simulink model "CircuitB_cbv_only"  (R2024b)
settings: Solver=VariableStepAuto  StartTime=0.0  StopTime=60  MaxStep=1e-3  RelTol=1e-3
InitFcn:
  | run("circuit_B.m")
model workspace (MATLAB code in the model file):
  | %% From Project Description
  | omega_0 = 5; % [rad/sec]
  | % eta_hmM = 1;
  | % eta_vM = 1; % 100% since parallel orifices simulate this
  | 
  | %% Chosen Parameters
  | 
  | wn = 17 * 2*pi; %from datasheet
  | zeta = 1;
  | 
  | dpO_CBV = 200e5;
  | dpO_CHK = 2e5; % default 2 MRH
  | dpO_comp = 3e5; % from 5 to 10, default 3 MRH
  | 
  | pCrCBV = 216e5;
  | pCrCHK = 1.7e5; % [bar] datasheet
  | pCMP = 10e5;
  | 
  | fCO = 2; % [Hz]
  | wCO = 2*pi * fCO; % [rad/sec]
  | 
  | % alpha = 3;
  | % pCrCHK = 2;
  | 
  | %% Calculated Parameters
undefined symbols (not defined in the file): Ad_L, Ad_L_fault, alpha_cbv, g, i_pl2M, mpl, mu_eq, pcr2, Tw, Zw
libraries: nesl_utility x19, fl_lib x19, SimscapeFluids_lib x13, slpidlib x2
(part 2 of 2)

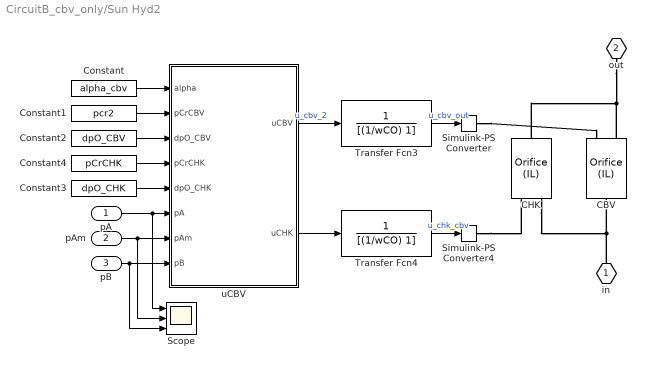
== system CircuitB_cbv_only/Sun Hyd2 ==
  pA : Inport
  pAm : Inport  Port=2
  pB : Inport  Port=3
  CBV : SimscapeFluids_lib/Isothermal Liquid/Valves & Orifices/Orifices/Orifice (IL)  orifice_type=foundation.enum.constant_variable.variable  constant_orifice_spec=fluids.isothermal_liquid.valves_orifices.orifices.enum.constant_orifice_spec.area  variable_orifice_spec=fluids.isothermal_liquid.valves_orifices.orifices.enum.orifice_spec.linear  orifice_area_constant=1e-3 m^2  p_diff_TLU_constant=[-4, -3, -2, -1, -.5, 0, .5, 1, 2, 3, 4] MPa  vol_flow_TLU_constant=[-2.44, -2.12, -1.68, -1.22, -.84, 0, .85, 1.21, 1.7, 2.09, 2.41] .* 1e-3 m^3/s  S_min=0 m  del_S=1 m  open_orientation=fluids.isothermal_liquid.valves_orifices.orifices.enum.orifice_orientation.positive  area_max=AdCBV m^2  area_leak=0.001 mm^2  S_TLU=[0, .002, .004, .007, .017] m  orifice_area_TLU=[1e-09, 2.0352e-07, 4.0736e-05, .00011438, .00034356] m^2  area=inf m^2  Cd=CdCBV  Re_c=150  smoothing_factor=0.01  pressure_recovery=false  S_vol_flow_TLU=[0, .002, .004, .007, .017] m  p_diff_TLU=[.3, .5, .7] MPa  vol_flow_TLU=1e-3 * [1.7e-05, 2e-05, 2.6e-05; .0035, .0045, .0053; .7, .9, 1.06; 1.96, 2.5, 3; 6, 7.7, 9.13] m^3/s
      settings: InternalSimscapePortConfiguration="{\"Bottom\":[],\"Left\":[{\"id\":\"A\",\"label\":\"A\",\"type\":\"foundation.isothermal_liquid.isothermal_liquid\"},{\"id\":\"S\",\"label\":\"S\",\"type\":\"input\"}],\"Right\":[{\"id\":\"B\",\"label\":\"B\",\"type\":\"foundation.isothermal_liquid.isothermal_liquid\"}],\"Top\":[]}"
  CHK : SimscapeFluids_lib/Isothermal Liquid/Valves & Orifices/Orifices/Orifice (IL)  orifice_type=foundation.enum.constant_variable.variable  constant_orifice_spec=fluids.isothermal_liquid.valves_orifices.orifices.enum.constant_orifice_spec.area  variable_orifice_spec=fluids.isothermal_liquid.valves_orifices.orifices.enum.orifice_spec.linear  orifice_area_constant=1e-3 m^2  p_diff_TLU_constant=[-4, -3, -2, -1, -.5, 0, .5, 1, 2, 3, 4] MPa  vol_flow_TLU_constant=[-2.44, -2.12, -1.68, -1.22, -.84, 0, .85, 1.21, 1.7, 2.09, 2.41] .* 1e-3 m^3/s  S_min=0 m  del_S=1 m  open_orientation=fluids.isothermal_liquid.valves_orifices.orifices.enum.orifice_orientation.positive  area_max=AdCHK m^2  area_leak=0.001 mm^2  S_TLU=[0, .002, .004, .007, .017] m  orifice_area_TLU=[1e-09, 2.0352e-07, 4.0736e-05, .00011438, .00034356] m^2  area=inf m^2  Cd=CdCHK  Re_c=150  smoothing_factor=0.01  pressure_recovery=false  S_vol_flow_TLU=[0, .002, .004, .007, .017] m  p_diff_TLU=[.3, .5, .7] MPa  vol_flow_TLU=1e-3 * [1.7e-05, 2e-05, 2.6e-05; .0035, .0045, .0053; .7, .9, 1.06; 1.96, 2.5, 3; 6, 7.7, 9.13] m^3/s
      settings: InternalSimscapePortConfiguration="{\"Bottom\":[],\"Left\":[{\"id\":\"A\",\"label\":\"A\",\"type\":\"foundation.isothermal_liquid.isothermal_liquid\"},{\"id\":\"S\",\"label\":\"S\",\"type\":\"input\"}],\"Right\":[{\"id\":\"B\",\"label\":\"B\",\"type\":\"foundation.isothermal_liquid.isothermal_liquid\"}],\"Top\":[]}"
  Constant : Constant  Value=alpha_cbv
  Constant1 : Constant  Value=pcr2
  Constant2 : Constant  Value=dpO_CBV
  Constant3 : Constant  Value=dpO_CHK
  Constant4 : Constant  Value=pCrCHK
  Scope : Scope  NumInputPorts=3
  Simulink-PS Converter : nesl_utility/Simulink-PS Converter  PhysicalDomain=network_engine_domain  SubClassName=ps_input  LeftPortType=input  RightPortType=output  PseudoPeriodic=off  Frequencies=[]  NoiseDistribution=none  NoiseParameters=[]  Unit=1  AffineConversion=off  FilteringAndDerivatives=filter  SimscapeFilterOrder=2  InputFilterTimeConstant=0.001  UdotUserProvided=0
  Simulink-PS Converter4 : nesl_utility/Simulink-PS Converter  PhysicalDomain=network_engine_domain  SubClassName=ps_input  LeftPortType=input  RightPortType=output  PseudoPeriodic=off  Frequencies=[]  NoiseDistribution=none  NoiseParameters=[]  Unit=1  AffineConversion=off  FilteringAndDerivatives=filter  SimscapeFilterOrder=2  InputFilterTimeConstant=0.001  UdotUserProvided=0
  Transfer Fcn3 : TransferFcn  Denominator=[(1/wCO) 1]
  Transfer Fcn4 : TransferFcn  Denominator=[(1/wCO) 1]
  uCBV : MATLAB Function  TreatAsAtomicUnit=on
  in : PMIOPort  Side=Right
  out : PMIOPort  Port=2  Side=Left
  wires:
  uCBV/1(uCBV) -> Transfer Fcn3/1  "u_cbv_2"
  Transfer Fcn3/1 -> Simulink-PS Converter/1  "u_cbv_out"
  pA/1 -> Scope/1, uCBV/6(pA)
  Transfer Fcn4/1 -> Simulink-PS Converter4/1  "u_chk_cbv"
  pAm/1 -> Scope/2, uCBV/7(pAm)
  uCBV/2(uCHK) -> Transfer Fcn4/1
  pB/1 -> Scope/3, uCBV/8(pB)
  Constant/1 -> uCBV/1(alpha)
  Constant1/1 -> uCBV/2(pCrCBV)
  Constant2/1 -> uCBV/3(dpO_CBV)
  Constant3/1 -> uCBV/5(dpO_CHK)
  Constant4/1 -> uCBV/4(pCrCHK)
  connections:
  CHK/RConn1 -- CBV/LConn1 -- out/RConn1
  CHK/LConn1 -- CBV/RConn1 -- in/RConn1
  Simulink-PS Converter4/RConn1 -- CHK/LConn2
  Simulink-PS Converter/RConn1 -- CBV/LConn2

== matlab function CircuitB_cbv_only/MATLAB Function1 ==
  data: zw input; Tw input; i_L2M input; t input; thetaRef output; thetaDotRef output
function [thetaRef,thetaDotRef] = referenceSignals(zw, Tw, i_L2M, t)

% Reference values for platform
zRef = zw * sin(2*pi/Tw * t); % [m]
zDotRef = 2*pi/Tw * zw * cos(2*pi/Tw * t); % [m/s]

% Reference values for motor
thetaRef = zRef/i_L2M; % [rad]
thetaDotRef = zDotRef/i_L2M; % [rad/sec]

% Envelope Functions
tEnv = 2*Tw; % [sec]
uEnv = t/tEnv; % [-]

if t < tEnv
    xEnv    = 3*uEnv^2    - 2*uEnv^3;
    xDotEnv = 6*uEnv/tEnv - 6*uEnv^2/tEnv;
else
    xEnv    = 1;
    xDotEnv = 0;
end

% Encorporating cubic polynomial into reference signals
thetaRef    = xEnv*thetaRef;
thetaDotRef = xEnv*thetaDotRef + xDotEnv*thetaRef;

== matlab function CircuitB_cbv_only/pumpRamp ==
  data: t input; p output; pPump input
function p = pumpRamp(t, pPump)

T = 0.2; % [sec]
tau = t/T; % [-]

if tau <= 1
    p = pPump*(3*tau^2 - 2*tau^3);
else
    p = pPump;
end

% p = 240e5;

== matlab function CircuitB_cbv_only/MATLAB Function ==
  data: AdLfault input; AdL input; s output; t input
function s = fcn(AdLfault, AdL, t)

% if t<= 30
    s = AdL/AdLfault;
% else
%     s = 1;
% end

== matlab function CircuitB_cbv_only/MATLAB Function3 ==
  data: MM0 input; MM output; mu_eq input; omega_0 input; omega_M input
function MM = motorMoment(MM0, mu_eq, omega_0, omega_M)

MM = MM0 * ( 1 + mu_eq * tanh(omega_M/omega_0) ); % [Nm]

== matlab function CircuitB_cbv_only/Compensator Valve/MATLAB Function2 ==
  data: pIN input; pLS input; uCMP output; dpO_comp input; pCMP input
function uCMP = cmp(pIN, pLS, dpO_comp, pCMP)

uCMP = (pLS + pCMP - pIN)/dpO_comp;

% Saturation
if uCMP > 1
    uCMP = 1;
elseif uCMP < 0
    uCMP = 0;
end

== matlab function CircuitB_cbv_only/Compensator Valve/pLS ==
  data: u input; pLS output; pA input; pB input
function pLS = fcn(u, pA, pB)

if u > 0
    pLS = pA;
else
    pLS = pB;
end

== matlab function CircuitB_cbv_only/Sun Hyd2/uCBV ==
  data: alpha input; pCrCBV input; dpO_CBV input; pCrCHK input; dpO_CHK input; uCBV output; pA input; pAm input; pB input; uCHK output
function [uCBV,uCHK] = fcn(alpha, pCrCBV, dpO_CBV, pCrCHK, dpO_CHK,pA, pAm, pB)

%%% CBV
uCBV = (alpha*pB + pAm - pCrCBV - (1 + alpha)*pA)/dpO_CBV;
    % Saturation
if uCBV > 1
    uCBV = 1;
elseif uCBV < 0
    uCBV = 0;
end

%%% Check Valve (CHK)
uCHK = (pA - pCrCHK - pAm)/dpO_CHK;
    % Saturation
if uCHK > 1
    uCHK = 1;
elseif uCHK < 0
    uCHK = 0;
end

== matlab function CircuitB_cbv_only/Sun Hyd1/uCBV ==
  data: alpha input; pCrCBV input; dpO_CBV input; pCrCHK input; dpO_CHK input; uCBV output; pA input; pAm input; pB input; uCHK output
function [uCBV,uCHK] = fcn(alpha, pCrCBV, dpO_CBV, pCrCHK, dpO_CHK,pA, pAm, pB)

%%% CBV
uCBV = (alpha*pB + pAm - pCrCBV - (1 + alpha)*pA)/dpO_CBV;
    % Saturation
if uCBV > 1
    uCBV = 1;
elseif uCBV < 0
    uCBV = 0;
end

%%% Check Valve (CHK)
uCHK = (pA - pCrCHK - pAm)/dpO_CHK;
    % Saturation
if uCHK > 1
    uCHK = 1;
elseif uCHK < 0
    uCHK = 0;
end
